simulink model "Embedded_control_motor_Full_EA_01"  (R2020b)
settings: Solver=FixedStepAuto  StartTime=0.0  StopTime=inf  FixedStep=0.2  RelTol=1e-3  EnableMultiTasking=on
undefined symbols (not defined in the file): DiscIntNeverNeededParam
libraries: arduinolib x10, simulink x3
settings Model: SILPILModeSetting=veronly  EnablePacing=on  ExtModeTrigDuration=2  Creator=Jezz  LastModifiedBy=Ege
settings OptimizationCC: EnhancedBackFolding=on  PassReuseOutputArgsAs=Individual arguments  ZeroExternalMemoryAtStartup=off  ZeroInternalMemoryAtStartup=off  MaxStackSize=64  OptimizeBlockOrder=speed  DifferentSizesBufferReuse=on  OptimizationCustomize=off  EfficientTunableParamExpr=on
settings DebuggingCC: ParameterTunabilityLossMsg=error
settings HardwareCC: ProdBitPerPointer=32  ProdBitPerSizeT=32  ProdBitPerPtrDiffT=32  ProdLargestAtomicInteger=Long  ProdLargestAtomicFloat=Double  ProdWordSize=32  ProdHWDeviceType=ARM Compatible->ARM Cortex
settings SFSimCC: MATLABDynamicMemAlloc=off
settings RTWCC: Description=Embedded Coder  SystemTargetFile=ert.tlc  HardwareBoard=Arduino Nano 33 IoT  TemplateMakefile=ert_default_tmf  Toolchain=Arduino ARM  BuildConfiguration=Faster Runs
settings CodeAppCC: ForceParamTrailComments=on  IgnoreCustomStorageClasses=off  OperatorAnnotations=on  SimulinkDataObjDesc=on  SFDataObjDesc=on  InsertBlockDesc=on
settings ERTTargetCC: SupportContinuousTime=on  SupportVariableSizeSignals=on  ExtModeTransport=3  ExtModeStaticAllocSize=8192  ExtModeMexFile=ext_xcp  ExtModeIntrfLevel=Level2 - Open

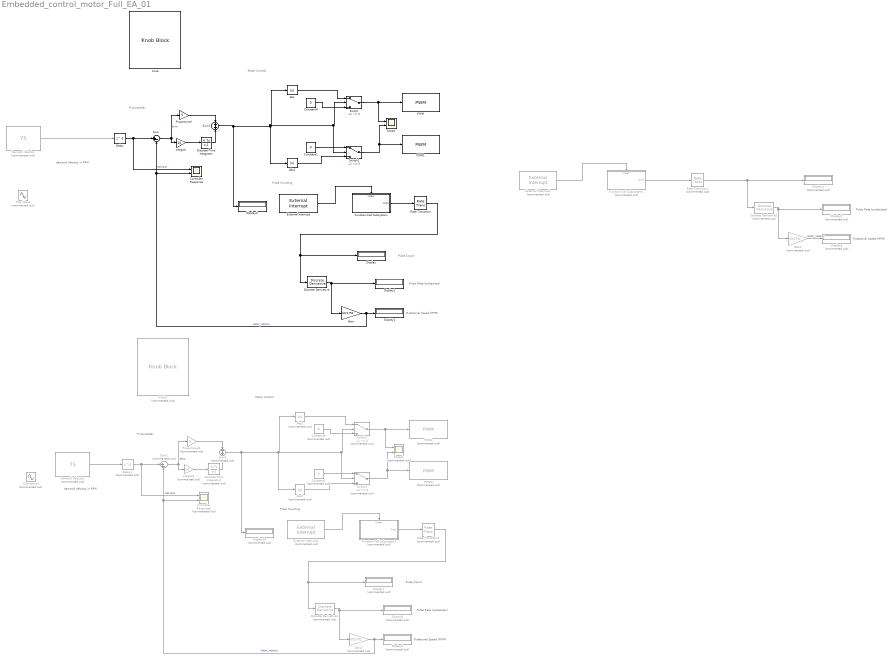
== system Embedded_control_motor_Full_EA_01 ==
  note: demand Velocity in RPM
  note: Pulse Counting
  note: Motor Control
  note: Pulse Rate (pulses/sec)
  note: Pulse Count
  note: Rotational Speed (RPM)
  note: PI Controller
  note: Rotational Speed (RPM)
  note: Pulse Rate (pulses/sec)
  note: Pulse Count
  note: Rotational Speed (RPM)
  note: Pulse Rate (pulses/sec)
  note: PI Controller
  note: Pulse Counting
  note: demand Velocity in RPM
  note: Motor Control
  Abs : Abs
  Abs1 : Abs
  Abs2 : Abs  Commented=on
  Abs3 : Abs  Commented=on
  Constant1 : Constant  Value=0  OutDataTypeStr=uint8  SampleTime=-1
  Constant2 : Constant  Commented=on  Value=0  OutDataTypeStr=uint8  SampleTime=-1
  Constant3 : Constant  Commented=on  Value=0  OutDataTypeStr=uint8  SampleTime=-1
  Constant4 : Constant  Value=0  OutDataTypeStr=uint8  SampleTime=-1
  Controller Response : Scope  NumInputPorts=2
  Controller Response1 : Scope  Commented=on  NumInputPorts=2
  Delay : Delay
  Delay1 : Delay  Commented=on
  Demand Velocity : Constant  Commented=on  Value=75
  Demand Velocity1 : Constant  Commented=on  Value=75
  Discrete Derivative : simulink/Discrete/Discrete Derivative  gainval=1.0  ICPrevScaledInput=0.0  OutMin=[]  OutMax=[]  OutDataType=fixdt(1, 16)  OutScaling=2^-10  DoSatur=off
  Discrete Derivative1 : simulink/Discrete/Discrete Derivative  Commented=on  gainval=1.0  ICPrevScaledInput=0.0  OutMin=[]  OutMax=[]  OutDataType=fixdt(1, 16)  OutScaling=2^-10  DoSatur=off
  Discrete Derivative2 : simulink/Discrete/Discrete Derivative  Commented=on  gainval=1.0  ICPrevScaledInput=0.0  OutMin=[]  OutMax=[]  OutDataType=fixdt(1, 16)  OutScaling=2^-10  DoSatur=off
  Discrete-Time Integrator : DiscreteIntegrator  SampleTime=-1  ICPrevOutput=DiscIntNeverNeededParam  ICPrevScaledInput=DiscIntNeverNeededParam
  Discrete-Time Integrator1 : DiscreteIntegrator  Commented=on  SampleTime=-1  ICPrevOutput=DiscIntNeverNeededParam  ICPrevScaledInput=DiscIntNeverNeededParam
  Display{,1..3} (4 alike) : Display
  Display{4..10} (7 alike) : Display  Commented=on
  External Interrupt : arduinolib/External Interrupt  Pin=2  PullUp=off  Mode=RISING  InterruptSimulationInput=off
      settings: SourceProductBaseCode=ARDUINO
  External Interrupt1 : arduinolib/External Interrupt  Commented=on  Pin=2  PullUp=off  Mode=RISING  InterruptSimulationInput=off
      settings: SourceProductBaseCode=ARDUINO
  External Interrupt2 : arduinolib/External Interrupt  Commented=on  Pin=15  PullUp=off  Mode=RISING  InterruptSimulationInput=off
      settings: SourceProductBaseCode=ARDUINO
  Function-Call Subsystem : Subsystem  TreatAsAtomicUnit=on
  Function-Call Subsystem1 : Subsystem  Commented=on  TreatAsAtomicUnit=on
  Function-Call Subsystem2 : Subsystem  Commented=on  TreatAsAtomicUnit=on
  Gain : Gain  Gain=60/1792
  Gain1 : Gain  Commented=on  Gain=60/1792
  Gain2 : Gain  Commented=on  Gain=60/1792
  Integral : Gain  Gain=10
  Integral1 : Gain  Commented=on  Gain=10
  Knob : KnobBlock  ScaleMax=75
  Knob1 : KnobBlock  Commented=on  ScaleMax=75
  PWM : arduinolib/PWM  pinNumber=10  frequencyType=Default  desiredFrequency=500  achievableFrequency=500
  PWM1 : arduinolib/PWM  pinNumber=11  frequencyType=Default  desiredFrequency=500  achievableFrequency=500
  PWM2 : arduinolib/PWM  Commented=on  pinNumber=6  frequencyType=Default  desiredFrequency=500  achievableFrequency=500
  PWM3 : arduinolib/PWM  Commented=on  pinNumber=9  frequencyType=Default  desiredFrequency=500  achievableFrequency=500
  Proportional : Gain  Gain=5
  Proportional1 : Gain  Commented=on  Gain=5
  Rate Transition : RateTransition  Deterministic=off
  Rate Transition1 : RateTransition  Commented=on  Deterministic=off
  Rate Transition2 : RateTransition  Commented=on  Deterministic=off
  Scope : Scope  NumInputPorts=2
  Scope1 : Scope  Commented=on  NumInputPorts=2
  Sine Wave : Sin  Commented=on  Amplitude=52  SampleTime=0
  Sine Wave1 : Sin  Commented=on  Amplitude=52  SampleTime=0
  Sum : Sum  Inputs=|+-
  Sum1 : Sum  Inputs=+|+
  Sum2 : Sum  Commented=on  Inputs=|+-
  Sum3 : Sum  Commented=on  Inputs=+|+
  Switch : Switch
  Switch1 : Switch
  Switch2 : Switch  Commented=on
  Switch3 : Switch  Commented=on
  wires:
  Abs/1 -> Switch/1
  Constant4/1 -> Switch/3
  Switch/1 -> Scope/1, PWM/1
  Abs1/1 -> Switch1/3
  Constant1/1 -> Switch1/1
  Switch1/1 -> PWM1/1, Scope/2
  Rate Transition/1 -> Discrete Derivative/1, Display/1
  External Interrupt/1 -> Function-Call Subsystem/Trigger
  Discrete Derivative/1 -> Gain/1, Display1/1
  Function-Call Subsystem/1(Out1) -> Rate Transition/1
  Discrete-Time Integrator/1 -> Sum1/2
  Integral/1 -> Discrete-Time Integrator/1
  Sum/1 -> Proportional/1, Integral/1  "Error"
  Delay/1 -> Controller Response/1, Sum/1  "Demand"
  Gain/1 -> Controller Response/2, Sum/2, Display2/1  "Motor_Velocity"
  Proportional/1 -> Sum1/1
  Sum1/1 -> Switch1/2, Switch/2, Abs/1, Abs1/1, Display3/1
  External Interrupt1/1 -> Function-Call Subsystem1/Trigger
  Function-Call Subsystem1/1(Out1) -> Rate Transition1/1
  Gain1/1 -> Display6/1  "Motor_Velocity"
  Rate Transition1/1 -> Discrete Derivative1/1, Display4/1
  Discrete Derivative1/1 -> Gain1/1, Display5/1
  Switch3/1 -> PWM3/1, Scope1/2
  Discrete-Time Integrator1/1 -> Sum3/2
  Sum2/1 -> Proportional1/1, Integral1/1  "Error"
  Proportional1/1 -> Sum3/1
  Sum3/1 -> Abs2/1, Switch2/2, Switch3/2, Abs3/1, Display10/1
  Constant3/1 -> Switch2/3
  Discrete Derivative2/1 -> Gain2/1, Display8/1
  Abs3/1 -> Switch3/3
  External Interrupt2/1 -> Function-Call Subsystem2/Trigger
  Switch2/1 -> Scope1/1, PWM2/1
  Delay1/1 -> Controller Response1/1, Sum2/1  "Demand"
  Function-Call Subsystem2/1(Out1) -> Rate Transition2/1
  Rate Transition2/1 -> Discrete Derivative2/1, Display7/1
  Constant2/1 -> Switch3/1
  Gain2/1 -> Controller Response1/2, Sum2/2, Display9/1  "Motor_Velocity"
  Abs2/1 -> Switch2/1
  Integral1/1 -> Discrete-Time Integrator1/1
  Demand Velocity1/1 -> Delay1/1
  Demand Velocity/1 -> Delay/1

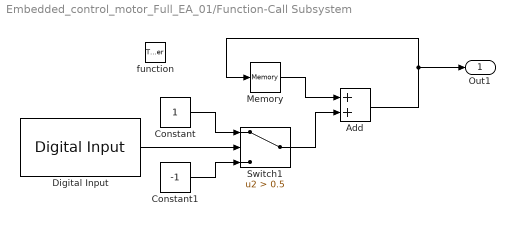
== system Embedded_control_motor_Full_EA_01/Function-Call Subsystem ==
  function : TriggerPort  TriggerType=function-call  VariantControl=Variant
  Add : Sum
  Constant : Constant  SampleTime=-1
  Constant1 : Constant  Value=-1  SampleTime=-1
  Digital Input : arduinolib/Digital Input  pinNumber=3  mode=Default  Direction=input  SampleTime=-1  blockPlatform=arduino
  Memory : Memory  InheritSampleTime=on
  Switch1 : Switch  Criteria=u2 > Threshold  Threshold=0.5
  Out1 : Outport
  wires:
  Constant/1 -> Switch1/1
  Memory/1 -> Add/1
  Add/1 -> Memory/1, Out1/1
  Digital Input/1 -> Switch1/2
  Constant1/1 -> Switch1/3
  Switch1/1 -> Add/2

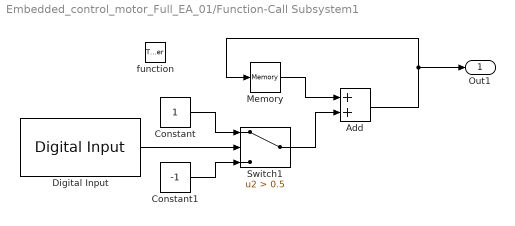
== system Embedded_control_motor_Full_EA_01/Function-Call Subsystem1 ==
  function : TriggerPort  TriggerType=function-call  VariantControl=Variant
  Add : Sum
  Constant : Constant  SampleTime=-1
  Constant1 : Constant  Value=-1  SampleTime=-1
  Digital Input : arduinolib/Digital Input  pinNumber=4  mode=Default  Direction=input  SampleTime=-1  blockPlatform=arduino
  Memory : Memory  InheritSampleTime=on
  Switch1 : Switch  Criteria=u2 > Threshold  Threshold=0.5
  Out1 : Outport
  wires:
  Constant/1 -> Switch1/1
  Memory/1 -> Add/1
  Add/1 -> Memory/1, Out1/1
  Digital Input/1 -> Switch1/2
  Constant1/1 -> Switch1/3
  Switch1/1 -> Add/2

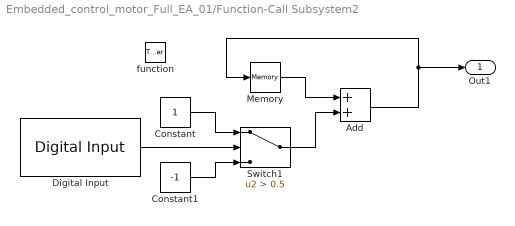
== system Embedded_control_motor_Full_EA_01/Function-Call Subsystem2 ==
  function : TriggerPort  TriggerType=function-call  VariantControl=Variant
  Add : Sum
  Constant : Constant  SampleTime=-1
  Constant1 : Constant  Value=-1  SampleTime=-1
  Digital Input : arduinolib/Digital Input  pinNumber=13  mode=Default  Direction=input  SampleTime=-1  blockPlatform=arduino
  Memory : Memory  InheritSampleTime=on
  Switch1 : Switch  Criteria=u2 > Threshold  Threshold=0.5
  Out1 : Outport
  wires:
  Constant/1 -> Switch1/1
  Memory/1 -> Add/1
  Add/1 -> Memory/1, Out1/1
  Digital Input/1 -> Switch1/2
  Constant1/1 -> Switch1/3
  Switch1/1 -> Add/2
